simulink model "mInterpolatedStateSpaceThermalModel_PassiveCooling"  (R2021b)
settings: Solver=VariableStepAuto  StartTime=0.0  StopTime=4000  FixedStep=0.2  RelTol=1e-3  AbsTol=1e-3
model workspace (MAT data in the model file):
  AdjacencyMat = [0 0 0 0 0 0 0 0 0 0 0 0 ... (22500 elements, 150x150)]
  Amat = [-2.52168311675e-20 0.000185215342392 0.000393846973431 9.92986102674e-12 0.00031646152302 0.000393854116246 9.92986102674e-12 0.000324664141987 1.81447431396e-13 1.18068931505e-12 1.12921110135e-12 5.64605550675e-13 ... (22500 elements, 150x150)]
  Bmat = [1e-20 0 0 0 0 0 0 0 0 0 0 0 ... (22500 elements, 150x150)]
  CapMat = [1e+20; 3424.01569452; 201.412687913; 100.706343957; 1759.15244838; 201.412687913; 100.706343957; 1759.15244838; 5511.23811622; 846.962860806; 885.574007203; 1771.14801441; 3602.91754031; 1285.19570945; 262.442367096; 96.4861643734; 524.884734191; 192.972328747; 1.6736656525; 1.6736656525; 197.840016; 146.536447734; 146.536447734; 514.702505759; 514.702505759; 1e+20; 0; 0; 0; 0; 0; 920.550315019; 0; 0; 0; 0; 0; 920.550315019; 0; 0; 0; 0; 0; 0; 1489.05793421; 0; 0; 0; 0; 189.651516828; 0; 0; 0; 0; 189.651516828; 0; 0; 0; 0; 0; 0; 274.797556911; 282.320953602; 0; 0; 0; 0; 189.651516828; 0; 0; 0; 0; 189.651516828; 0; 0; 0; 0; 0; 274.797556911; 282.320953602; 0; 0; 0; 0; 189.651516828; 0; 0; 0; 0; 189.651516828; 0; 0; 0; 0; 0; 274.797556911; 282.320953602; 0; 0; 0; 0; 178.512838093; 0; 0; 0; 0; 178.512838093; 0; 0; 0; 0; 0; 258.658051386; 282.320953602; 0; 0; 0; 0; 94.8257584142; 0; 0; 0; 0; 94.8257584142; 0; 0; 0; 0; 0; 137.398778455; 282.320953602; 0; 0; 0; 0; 0; 94.8257584142; 0; 0; 0; 0; 0; 94.8257584142; 0; 0; 0; 0; 0; 137.398778455; 282.320953602]
  CoolantArrayIdxs = [21; 26]
  CoolantNodeIdxs = [21; 26]
  Friction_Loss_Mat = [0  0  0  0  0  0  0  0  0  0; 0  0  0  0  0  0  0  0  0  0; 0  0  0  0  0  0  0  0  0  0; 0  0  0  0  0  0  0  0  0  0; 0  0  0  0  0  0  0  0  0  0; 0  0  0  0  0  0  0  0  0  0; 0  0  0  0  0  0  0  0  0  0; 0  0  0  0  0  0  0  0  0  0; 0  0  0  0  0  0  0  0  0  0; 0  0  0  0  0  0  0  0  0  0; 0  0  0  0  0  0  0  0  0  0; 0  0  0  0  0  0  0  0  0  0; 0  0  0  0  0  0  0  0  0  0; 0  0  0  0  0  0  0  0  0  0; 0  0  0  0  0  0  0  0  0  0; 0  0  0  0  0  0  0  0  0  0; 0  0  0  0  0  0  0  0  0  0; 0  0  0  0  0  0  0  0  0  0; 0  0  0  0  0  0  0  0  0  0; 0  0  0  0  0  0  0  0  0  0; 0  0  0  0  0  0  0  0  0  0; 0  0  0  0  0  0  0  0  0  0; 0  0  0  0  0  0  0  0  0  0; 0  0  0  0  0  0  0  0  0  0; 0  0  0  0  0  0  0  0  0  0; 0  0  0  0  0  0  0  0  0  0; 0  0  0  0  0  0  0  0  0  0; 0  0  0  0  0  0  0  0  0  0; 0  0  0  0  0  0  0  0  0  0; 0  0  0  0  0  0  0  0  0  0; 0  0  0  0  0  0  0  0  0  0; 0  0  0  0  0  0  0  0  0  0; 0  0  0  0  0  0  0  0  0  0; 0  0  0  0  0  0  0  0  0  0; 0  0  0  0  0  0  0  0  0  0; 0  0  0  0  0  0  0  0  0  0; 0  0  0  0  0  0  0  0  0  0; 0  0  0  0  0  0  0  0  0  0; 0  0  0  0  0  0  0  0  0  0; 0  0  0  0  0  0  0  0  0  0; 0  0  0  0  0  0  0  0  0  0; 0  0  0  0  0  0  0  0  0  0; 0  0  0  0  0  0  0  0  0  0; 0  0  0  0  0  0  0  0  0  0; 0  0  0  0  0  0  0  0  0  0; 0  0  0  0  0  0  0  0  0  0; 0  0  0  0  0  0  0  0  0  0; 0  0  0  0  0  0  0  0  0  0; 0  0  0  0  0  0  0  0  0  0; 0  0  0  0  0  0  0  0  0  0; 0  0  0  0  0  0  0  0  0  0; 0  0  0  0  0  0  0  0  0  0; 0  0  0  0  0  0  0  0  0  0; 0  0  0  0  0  0  0  0  0  0; 0  0  0  0  0  0  0  0  0  0; 0  0  0  0  0  0  0  0  0  0; 0  0  0  0  0  0  0  0  0  0; 0  0  0  0  0  0  0  0  0  0; 0  0  0  0  0  0  0  0  0  0; 0  0  0  0  0  0  0  0  0  0]
  InletCoolIdxs = 26
  Iron_Loss_Rotor_Back_Iron_Mat = [5.88721488028e-06 1.56097290893e-05 2.53322432983e-05 3.50547575073e-05 4.22932634361e-05 4.83272215068e-05 5.43611795774e-05 6.0395137648e-05 6.64290957187e-05 7.24630537893e-05 7.84507163281e-05 8.35639993023e-05 ... (600 elements, 60x10)]
  Iron_Loss_Rotor_Pole_Mat = [0  0  0  0  0  0  0  0  0  0; 0  0  0  0  0  0  0  0  0  0; 0  0  0  0  0  0  0  0  0  0; 0  0  0  0  0  0  0  0  0  0; 0  0  0  0  0  0  0  0  0  0; 0  0  0  0  0  0  0  0  0  0; 0  0  0  0  0  0  0  0  0  0; 0  0  0  0  0  0  0  0  0  0; 0  0  0  0  0  0  0  0  0  0; 0  0  0  0  0  0  0  0  0  0; 0  0  0  0  0  0  0  0  0  0; 0  0  0  0  0  0  0  0  0  0; 0  0  0  0  0  0  0  0  0  0; 0  0  0  0  0  0  0  0  0  0; 0  0  0  0  0  0  0  0  0  0; 0  0  0  0  0  0  0  0  0  0; 0  0  0  0  0  0  0  0  0  0; 0  0  0  0  0  0  0  0  0  0; 0  0  0  0  0  0  0  0  0  0; 0  0  0  0  0  0  0  0  0  0; 0  0  0  0  0  0  0  0  0  0; 0  0  0  0  0  0  0  0  0  0; 0  0  0  0  0  0  0  0  0  0; 0  0  0  0  0  0  0  0  0  0; 0  0  0  0  0  0  0  0  0  0; 0  0  0  0  0  0  0  0  0  0; 0  0  0  0  0  0  0  0  0  0; 0  0  0  0  0  0  0  0  0  0; 0  0  0  0  0  0  0  0  0  0; 0  0  0  0  0  0  0  0  0  0; 0  0  0  0  0  0  0  0  0  0; 0  0  0  0  0  0  0  0  0  0; 0  0  0  0  0  0  0  0  0  0; 0  0  0  0  0  0  0  0  0  0; 0  0  0  0  0  0  0  0  0  0; 0  0  0  0  0  0  0  0  0  0; 0  0  0  0  0  0  0  0  0  0; 0  0  0  0  0  0  0  0  0  0; 0  0  0  0  0  0  0  0  0  0; 0  0  0  0  0  0  0  0  0  0; 0  0  0  0  0  0  0  0  0  0; 0  0  0  0  0  0  0  0  0  0; 0  0  0  0  0  0  0  0  0  0; 0  0  0  0  0  0  0  0  0  0; 0  0  0  0  0  0  0  0  0  0; 0  0  0  0  0  0  0  0  0  0; 0  0  0  0  0  0  0  0  0  0; 0  0  0  0  0  0  0  0  0  0; 0  0  0  0  0  0  0  0  0  0; 0  0  0  0  0  0  0  0  0  0; 0  0  0  0  0  0  0  0  0  0; 0  0  0  0  0  0  0  0  0  0; 0  0  0  0  0  0  0  0  0  0; 0  0  0  0  0  0  0  0  0  0; 0  0  0  0  0  0  0  0  0  0; 0  0  0  0  0  0  0  0  0  0; 0  0  0  0  0  0  0  0  0  0; 0  0  0  0  0  0  0  0  0  0; 0  0  0  0  0  0  0  0  0  0; 0  0  0  0  0  0  0  0  0  0]
  Iron_Loss_Rotor_Tooth_Mat = [0.0278606638652 0.0738715035935 0.119882343322 0.16589318305 0.184288576483 0.189292659205 0.194296741928 0.19930082465 0.204304907373 0.209308990095 0.214192013795 0.216788606579 ... (600 elements, 60x10)]
  Iron_Loss_Stator_Back_Iron_Mat = [0.538257512426 1.42720259745 2.31614768248 3.2050927675 3.70144029641 4.00740901333 4.31337773026 4.61934644718 4.9253151641 5.23128388103 5.53405994351 5.77653662762 ... (600 elements, 60x10)]
  Iron_Loss_Stator_Tooth_Mat = [0.271379868831 0.719570446697 1.16776102456 1.61595160243 1.84620127177 1.97076681088 2.09533234999 2.2198978891 2.34446342821 2.46902896732 2.59210855121 2.687123032 ... (600 elements, 60x10)]
  LossDistrForEachType = [0 0 0 0 0 0 0 0 0 0 0 0 ... (2400 elements, 16x150)]
  Magnet_Loss_Mat = [0  0  0  0  0  0  0  0  0  0; 0  0  0  0  0  0  0  0  0  0; 0  0  0  0  0  0  0  0  0  0; 0  0  0  0  0  0  0  0  0  0; 0  0  0  0  0  0  0  0  0  0; 0  0  0  0  0  0  0  0  0  0; 0  0  0  0  0  0  0  0  0  0; 0  0  0  0  0  0  0  0  0  0; 0  0  0  0  0  0  0  0  0  0; 0  0  0  0  0  0  0  0  0  0; 0  0  0  0  0  0  0  0  0  0; 0  0  0  0  0  0  0  0  0  0; 0  0  0  0  0  0  0  0  0  0; 0  0  0  0  0  0  0  0  0  0; 0  0  0  0  0  0  0  0  0  0; 0  0  0  0  0  0  0  0  0  0; 0  0  0  0  0  0  0  0  0  0; 0  0  0  0  0  0  0  0  0  0; 0  0  0  0  0  0  0  0  0  0; 0  0  0  0  0  0  0  0  0  0; 0  0  0  0  0  0  0  0  0  0; 0  0  0  0  0  0  0  0  0  0; 0  0  0  0  0  0  0  0  0  0; 0  0  0  0  0  0  0  0  0  0; 0  0  0  0  0  0  0  0  0  0; 0  0  0  0  0  0  0  0  0  0; 0  0  0  0  0  0  0  0  0  0; 0  0  0  0  0  0  0  0  0  0; 0  0  0  0  0  0  0  0  0  0; 0  0  0  0  0  0  0  0  0  0; 0  0  0  0  0  0  0  0  0  0; 0  0  0  0  0  0  0  0  0  0; 0  0  0  0  0  0  0  0  0  0; 0  0  0  0  0  0  0  0  0  0; 0  0  0  0  0  0  0  0  0  0; 0  0  0  0  0  0  0  0  0  0; 0  0  0  0  0  0  0  0  0  0; 0  0  0  0  0  0  0  0  0  0; 0  0  0  0  0  0  0  0  0  0; 0  0  0  0  0  0  0  0  0  0; 0  0  0  0  0  0  0  0  0  0; 0  0  0  0  0  0  0  0  0  0; 0  0  0  0  0  0  0  0  0  0; 0  0  0  0  0  0  0  0  0  0; 0  0  0  0  0  0  0  0  0  0; 0  0  0  0  0  0  0  0  0  0; 0  0  0  0  0  0  0  0  0  0; 0  0  0  0  0  0  0  0  0  0; 0  0  0  0  0  0  0  0  0  0; 0  0  0  0  0  0  0  0  0  0; 0  0  0  0  0  0  0  0  0  0; 0  0  0  0  0  0  0  0  0  0; 0  0  0  0  0  0  0  0  0  0; 0  0  0  0  0  0  0  0  0  0; 0  0  0  0  0  0  0  0  0  0; 0  0  0  0  0  0  0  0  0  0; 0  0  0  0  0  0  0  0  0  0; 0  0  0  0  0  0  0  0  0  0; 0  0  0  0  0  0  0  0  0  0; 0  0  0  0  0  0  0  0  0  0]
  OutletCoolIdxs = 21
  RotorCopperTempCoefResistivity = 0.00393
  Rotor_Cage_Loss_Mat = [0.452081247683 6.23621443388 12.0203476201 17.8044808063 27.0746990775 38.0353933249 48.9960875724 59.9567818198 70.9174760673 81.8781703148 93.2562227653 112.516882212 ... (600 elements, 60x10)]
  ShaftTorqueVec = [0.50751379462 6.70424518063 12.9009765666 19.0977079526 25.2944393387 31.4911707247 37.6879021107 43.8846334967 50.0813648827 56.2780962687 62.4748276547 68.6715590407 74.8682904267 81.0650218127 87.2617531987 93.4584845847 99.6552159708 105.851947357 112.048678743 118.245410129 124.442141515 130.638872901 136.835604287 143.032335673 149.229067059 155.425798445 161.622529831 167.819261217 174.015992603 180.212723989 186.409455375 192.606186761 198.802918147 204.999649533 211.196380919 217.393112305 223.589843691 229.786575077 235.983306463 242.180037849 248.376769235 254.573500621 260.770232007 266.966963393 273.163694779 279.360426165 285.557157551 291.753888937 297.950620323 304.147351709 310.344083095 316.540814481 322.737545867 328.934277253 335.131008639 341.327740025 347.524471411 353.721202797 359.917934183 366.114665569]
  Sig = Simulink.Signal
  Sig.DataType = 'auto'
  Sig.Dimensions = -1
  Sig.DimensionsMode = 'auto'
  Sig.Complexity = 'auto'
  Sig.SampleTime = -1
  Sig.SamplingMode = 'auto'
  SpeedVec = [200 1511.11111111 2822.22222222 4133.33333333 5444.44444444 6755.55555556 8066.66666667 9377.77777778 10688.8888889 12000]
  StateSpaceND : object (value not decoded)
  StatorCopperTempCoefResistivity = 0.00393
  Stator_Copper_Loss_Mat = [2.8235353719 37.2375386139 71.6515418559 106.065545098 145.96632659 188.527762252 231.089197915 273.650633577 316.212069239 358.773504901 402.558474022 469.452209983 ... (600 elements, 60x10)]
  Stray_Load_Loss_Mat = [0.107367111702 1.41831699713 2.72926688255 4.04021676798 5.3511666534 6.66211653882 7.97306642425 9.28401630967 10.5949661951 11.9059160805 13.2168659659 14.5278158514 ... (600 elements, 60x10)]
  Stray_Loss_Stator_Iron_Proportion = 0.95
  TinVal = 20
  TnodesInit = [20; 20; 20; 20; 20; 20; 20; 20; 20; 20; 20; 20; 20; 20; 20; 20; 20; 20; 20; 20; 20; 20; 20; 20; 20; 20; 20; 20; 20; 20; 20; 20; 20; 20; 20; 20; 20; 20; 20; 20; 20; 20; 20; 20; 20; 20; 20; 20; 20; 20; 20; 20; 20; 20; 20; 20; 20; 20; 20; 20; 20; 20; 20; 20; 20; 20; 20; 20; 20; 20; 20; 20; 20; 20; 20; 20; 20; 20; 20; 20; 20; 20; 20; 20; 20; 20; 20; 20; 20; 20; 20; 20; 20; 20; 20; 20; 20; 20; 20; 20; 20; 20; 20; 20; 20; 20; 20; 20; 20; 20; 20; 20; 20; 20; 20; 20; 20; 20; 20; 20; 20; 20; 20; 20; 20; 20; 20; 20; 20; 20; 20; 20; 20; 20; 20; 20; 20; 20; 20; 20; 20; 20; 20; 20; 20; 20; 20; 20; 20; 20]
  TrefRotor = 140
  TrefStator = 100
  TrotorRef = 140
  TwindingRef = 100
  Windage_Loss_Mat = [0  0  0  0  0  0  0  0  0  0; 0  0  0  0  0  0  0  0  0  0; 0  0  0  0  0  0  0  0  0  0; 0  0  0  0  0  0  0  0  0  0; 0  0  0  0  0  0  0  0  0  0; 0  0  0  0  0  0  0  0  0  0; 0  0  0  0  0  0  0  0  0  0; 0  0  0  0  0  0  0  0  0  0; 0  0  0  0  0  0  0  0  0  0; 0  0  0  0  0  0  0  0  0  0; 0  0  0  0  0  0  0  0  0  0; 0  0  0  0  0  0  0  0  0  0; 0  0  0  0  0  0  0  0  0  0; 0  0  0  0  0  0  0  0  0  0; 0  0  0  0  0  0  0  0  0  0; 0  0  0  0  0  0  0  0  0  0; 0  0  0  0  0  0  0  0  0  0; 0  0  0  0  0  0  0  0  0  0; 0  0  0  0  0  0  0  0  0  0; 0  0  0  0  0  0  0  0  0  0; 0  0  0  0  0  0  0  0  0  0; 0  0  0  0  0  0  0  0  0  0; 0  0  0  0  0  0  0  0  0  0; 0  0  0  0  0  0  0  0  0  0; 0  0  0  0  0  0  0  0  0  0; 0  0  0  0  0  0  0  0  0  0; 0  0  0  0  0  0  0  0  0  0; 0  0  0  0  0  0  0  0  0  0; 0  0  0  0  0  0  0  0  0  0; 0  0  0  0  0  0  0  0  0  0; 0  0  0  0  0  0  0  0  0  0; 0  0  0  0  0  0  0  0  0  0; 0  0  0  0  0  0  0  0  0  0; 0  0  0  0  0  0  0  0  0  0; 0  0  0  0  0  0  0  0  0  0; 0  0  0  0  0  0  0  0  0  0; 0  0  0  0  0  0  0  0  0  0; 0  0  0  0  0  0  0  0  0  0; 0  0  0  0  0  0  0  0  0  0; 0  0  0  0  0  0  0  0  0  0; 0  0  0  0  0  0  0  0  0  0; 0  0  0  0  0  0  0  0  0  0; 0  0  0  0  0  0  0  0  0  0; 0  0  0  0  0  0  0  0  0  0; 0  0  0  0  0  0  0  0  0  0; 0  0  0  0  0  0  0  0  0  0; 0  0  0  0  0  0  0  0  0  0; 0  0  0  0  0  0  0  0  0  0; 0  0  0  0  0  0  0  0  0  0; 0  0  0  0  0  0  0  0  0  0; 0  0  0  0  0  0  0  0  0  0; 0  0  0  0  0  0  0  0  0  0; 0  0  0  0  0  0  0  0  0  0; 0  0  0  0  0  0  0  0  0  0; 0  0  0  0  0  0  0  0  0  0; 0  0  0  0  0  0  0  0  0  0; 0  0  0  0  0  0  0  0  0  0; 0  0  0  0  0  0  0  0  0  0; 0  0  0  0  0  0  0  0  0  0; 0  0  0  0  0  0  0  0  0  0]
  flowrateVal = 5
  lossDistrEachType = [0 0 0 0 0 0 0 0 0 0 0 0 ... (2400 elements, 16x150)]
  lossEachTypeVal = [30; 30; 30; 30; 30; 30; 30; 30; 30; 30; 30; 30; 30; 30; 30; 30]
  nodelossVal = [1; 1; 1; 1; 1; 1; 1; 1; 1; 1; 1; 1; 1; 1; 1; 1; 1; 1; 1; 1; 1; 1; 1; 1; 1; 1; 1; 1; 1; 1; 1; 1; 1; 1; 1; 1; 1; 1; 1; 1; 1; 1; 1; 1; 1; 1; 1; 1; 1; 1; 1; 1; 1; 1; 1; 1; 1; 1; 1; 1; 1; 1; 1; 1; 1; 1; 1; 1; 1; 1; 1; 1; 1; 1; 1; 1; 1; 1; 1; 1; 1; 1; 1; 1; 1; 1; 1; 1; 1; 1; 1; 1; 1; 1; 1; 1; 1; 1; 1; 1; 1; 1; 1; 1; 1; 1; 1; 1; 1; 1; 1; 1; 1; 1; 1; 1; 1; 1; 1; 1; 1; 1; 1; 1; 1; 1; 1; 1; 1; 1; 1; 1; 1; 1; 1; 1; 1; 1; 1; 1; 1; 1; 1; 1; 1; 1; 1; 1; 1; 1]
  rotorCopperTempCoeff = 0.00393
  speedVal = 4000
  statorCopperTempCoeff = 0.00393
  torqueVal = 30
libraries: mcadROM_lib x1
settings Model: Creator=agonzale  LastModifiedBy=agonzale
settings SolverCC: AutoScaleAbsTol=off  NumberNewtonIterations=3

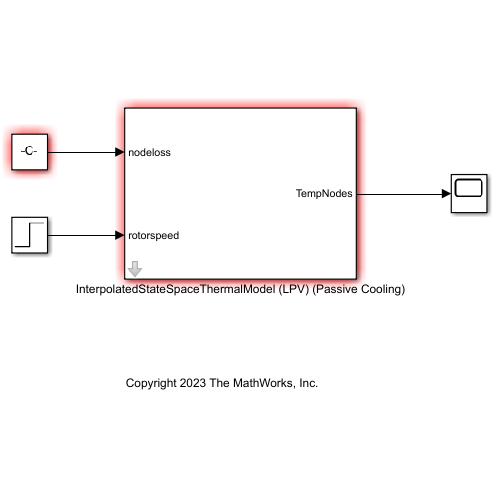
[thumbnail: Simulink's stored preview of the top-level diagram]
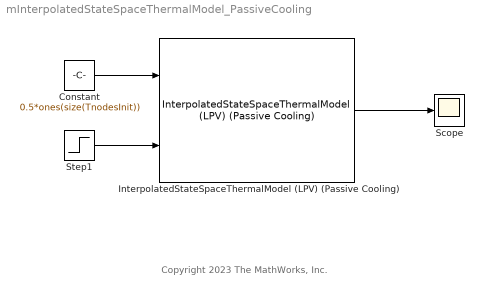
== system mInterpolatedStateSpaceThermalModel_PassiveCooling ==
  note: Copyright 2023 The MathWorks, Inc.
  Constant : Constant  Value=0.5*ones(size(TnodesInit))
  InterpolatedStateSpaceThermalModel (LPV) (Passive Cooling) : mcadROM_lib/InterpolatedStateSpaceThermalModel (LPV) (Passive Cooling)  StateSpaceND=StateSpaceND  TnodesInit=TnodesInit
  Scope : Scope
  Step1 : Step  Time=500  Before=1000  After=3000  SampleTime=0
  wires:
  Constant/1 -> InterpolatedStateSpaceThermalModel (LPV) (Passive Cooling)/1
  Step1/1 -> InterpolatedStateSpaceThermalModel (LPV) (Passive Cooling)/2
  InterpolatedStateSpaceThermalModel (LPV) (Passive Cooling)/1 -> Scope/1
